simulink model "GPI1"  (Simulink 7.0)
settings: Solver=ode45  StartTime=0.0  StopTime=1000.0  RelTol=1e-3
values from neighbouring files (symbols this model uses):
  A_gpegpi = 1    [data_GPE.m]    (also in data_GPI.m)
  A_gpi = 2    [data_GPI.m]
  A_stngpi = 1    [data_GPI.m]    (also in data_STN.m)
  B_gpegpi = .1    (= 0.1)    [data_GPE.m]    (also in data_GPI.m)
  B_gpi = .08    (= 0.08)    [data_GPI.m]
  B_stngpi = .05    (= 0.05)    [data_GPI.m]    (also in data_STN.m)
  c_gpi = 1    [data_GPI.m]
  cagi0 = i_v_16(289:304)    [launch_sysGPI_mod.m]
  egpegpi = -100    [data_synapses.m]
  ek_gpi = -80.0    (= -80)    [data_GPI.m]
  el_gpi = -55.0    (= -55)    [data_GPI.m]
  epsil_gpi = 1*10^-4    (= 0.0001)    [data_GPI.m]
  estngpi = 0    [data_synapses.m]
  gahp_gpi = 30.0    (= 30)    [data_GPI.m]
  gca_gpi = 0.15    [data_GPI.m]
  ggpegpi = ggpegpi_vec(i)    [CN_launch_CN_analyze_TAL2.m]    (also in data_synapses.m = 1; launch_sysGPI_mod.m = 0.3)
  gk_gpi = 30.0    (= 30)    [data_GPI.m]
  gl_gpi = .1    (= 0.1)    [data_GPI.m]
  gna_gpi = 120    [data_GPI.m]
  gstngpi = .3    (= 0.3)    [data_synapses.m]
  gt_gpi = .5    (= 0.5)    [data_GPI.m]
  hgi0 = i_v_16(241:256)    [launch_sysGPI_mod.m]
  k1_gpi = 30.0    (= 30)    [data_GPI.m]
  kca_gpi = 15    [data_GPI.m]
  ngi0 = i_v_16(257:272)    [launch_sysGPI_mod.m]
  phih_gpi = 0.05    [data_GPI.m]
  phin_gpi = 0.1    [data_GPI.m]
  phir_gpi = 1    [data_GPI.m]
  rgi0 = i_v_16(273:288)    [launch_sysGPI_mod.m]
  sgi0 = i_v_16(305:320)    [launch_sysGPI_mod.m]
  sig0 = i_v_16(209:224)    [launch_sysGPI_mod.m]
  sigmaa_gpi = 2    [data_GPI.m]
  sigmagh_gpe = 2.0    (= 2)    [data_GPE.m]
  sigmagh_gpi = 2.0    (= 2)    [data_GPI.m]
  sigmagh_stn = 8.0    (= 8)    [data_STN.m]
  sigmah_gpi = -12    [data_GPI.m]
  sigmam_gpi = 10.0    (= 10)    [data_GPI.m]
  sigman_gpi = 14.0    (= 14)    [data_GPI.m]
  sigmar_gpi = -2.0    (= -2)    [data_GPI.m]
  sigmas_gpi = 2    [data_GPI.m]
  sigmatauh_gpi = -12    [data_GPI.m]
  sigmataun_gpi = -12.0    (= -12)    [data_GPI.m]
  sis0 = i_v_16(97:112)    [launch_sysGPI_mod.m]
  tauh0_gpi = .05    (= 0.05)    [data_GPI.m]
  tauh1_gpi = .27    (= 0.27)    [data_GPI.m]
  taun0_gpi = .05    (= 0.05)    [data_GPI.m]
  taun1_gpi = .27    (= 0.27)    [data_GPI.m]
  taur_gpi = 30.0    (= 30)    [data_GPI.m]
  theta_gpe = 20    [data_GPE.m]    (also in data_GPI.m)
  theta_gpi = 20    [data_GPI.m]
  theta_stn = 30    [data_GPI.m]    (also in data_STN.m)
  thetaa_gpi = -57.0    (= -57)    [data_GPI.m]
  thetagh_gpe = -57.0    (= -57)    [data_GPE.m]
  thetagh_gpi = -57.0    (= -57)    [data_GPI.m]
  thetagh_stn = -39.0    (= -39)    [data_STN.m]
  thetah_gpi = -58.0    (= -58)    [data_GPI.m]
  thetam_gpi = -37.0    (= -37)    [data_GPI.m]
  thetan_gpi = -50.0    (= -50)    [data_GPI.m]
  thetar_gpi = -70.0    (= -70)    [data_GPI.m]
  thetas_gpi = -35.0    (= -35)    [data_GPI.m]
  thetatauh_gpi = -40.0    (= -40)    [data_GPI.m]
  thetataun_gpi = -40.0    (= -40)    [data_GPI.m]
  vgi0 = i_v_16(225:240)    [launch_sysGPI_mod.m]
(part 2 of 6)

== system GPI1/gpicomp1/syn_gpegpi ==
  In1 : Inport  OutDataType=sfix(16)  OutScaling=2^0
  In2 : Inport  Port=2  OutDataType=sfix(16)  OutScaling=2^0
  Fcn : Fcn  Expr=1/(1+exp(-(u-theta_gpe-thetagh_gpe)/sigmagh_gpe))
  Fcn2 : Fcn  Orientation=left  Expr=A_gpegpi*(1-u)
  Gain : Gain  Orientation=left  Gain=B_gpegpi  ParameterDataType=sfix(16)  ParameterScaling=2^0  OutDataType=sfix(16)  OutScaling=2^0  SaturateOnIntegerOverflow=on
  Integrator : Integrator  InitialConditionSource=external
  Product : Product  OutDataType=sfix(16)  OutScaling=2^0  SaturateOnIntegerOverflow=on  InputSameDT=on
  Sum : Sum  Inputs=|+-  OutDataType=sfix(16)  OutScaling=2^0  SaturateOnIntegerOverflow=on  InputSameDT=on
  Out1 : Outport  OutDataType=sfix(16)  OutScaling=2^0
  wires:
  Fcn/1 -> Product/1
  Fcn2/1 -> Product/2
  Product/1 -> Sum/1
  Sum/1 -> Integrator/1
  Integrator/1 -> Gain/1, Fcn2/1, Out1/1
  Gain/1 -> Sum/2
  In1/1 -> Fcn/1
  In2/1 -> Integrator/2

== system GPI1/gpicomp1/syn_gpegpi1 ==
  In1 : Inport  OutDataType=sfix(16)  OutScaling=2^0
  In2 : Inport  Port=2  OutDataType=sfix(16)  OutScaling=2^0
  Fcn : Fcn  Expr=1/(1+exp(-(u-theta_gpi-thetagh_gpi)/sigmagh_gpi))
  Fcn2 : Fcn  Orientation=left  Expr=A_gpi*(1-u)
  Gain : Gain  Orientation=left  Gain=B_gpi  ParameterDataType=sfix(16)  ParameterScaling=2^0  OutDataType=sfix(16)  OutScaling=2^0  SaturateOnIntegerOverflow=on
  Integrator : Integrator  InitialConditionSource=external
  Product : Product  OutDataType=sfix(16)  OutScaling=2^0  SaturateOnIntegerOverflow=on  InputSameDT=on
  Sum : Sum  Inputs=|+-  OutDataType=sfix(16)  OutScaling=2^0  SaturateOnIntegerOverflow=on  InputSameDT=on
  Out1 : Outport  OutDataType=sfix(16)  OutScaling=2^0
  wires:
  Fcn/1 -> Product/1
  Fcn2/1 -> Product/2
  Product/1 -> Sum/1
  Sum/1 -> Integrator/1
  Integrator/1 -> Gain/1, Fcn2/1, Out1/1
  Gain/1 -> Sum/2
  In1/1 -> Fcn/1
  In2/1 -> Integrator/2

== system GPI1/gpicomp1/syn_stngpi ==
  In1 : Inport  OutDataType=sfix(16)  OutScaling=2^0
  In2 : Inport  Port=2  OutDataType=sfix(16)  OutScaling=2^0
  Fcn : Fcn  Expr=1/(1+exp(-(u-theta_stn-thetagh_stn)/sigmagh_stn))
  Fcn2 : Fcn  Orientation=left  Expr=A_stngpi*(1-u)
  Gain : Gain  Orientation=left  Gain=B_stngpi  ParameterDataType=sfix(16)  ParameterScaling=2^0  OutDataType=sfix(16)  OutScaling=2^0  SaturateOnIntegerOverflow=on
  Integrator : Integrator  InitialConditionSource=external
  Product : Product  OutDataType=sfix(16)  OutScaling=2^0  SaturateOnIntegerOverflow=on  InputSameDT=on
  Sum : Sum  Inputs=|+-  OutDataType=sfix(16)  OutScaling=2^0  SaturateOnIntegerOverflow=on  InputSameDT=on
  Out1 : Outport  OutDataType=sfix(16)  OutScaling=2^0
  wires:
  Fcn/1 -> Product/1
  Fcn2/1 -> Product/2
  Product/1 -> Sum/1
  Sum/1 -> Integrator/1
  Integrator/1 -> Gain/1, Fcn2/1, Out1/1
  Gain/1 -> Sum/2
  In1/1 -> Fcn/1
  In2/1 -> Integrator/2

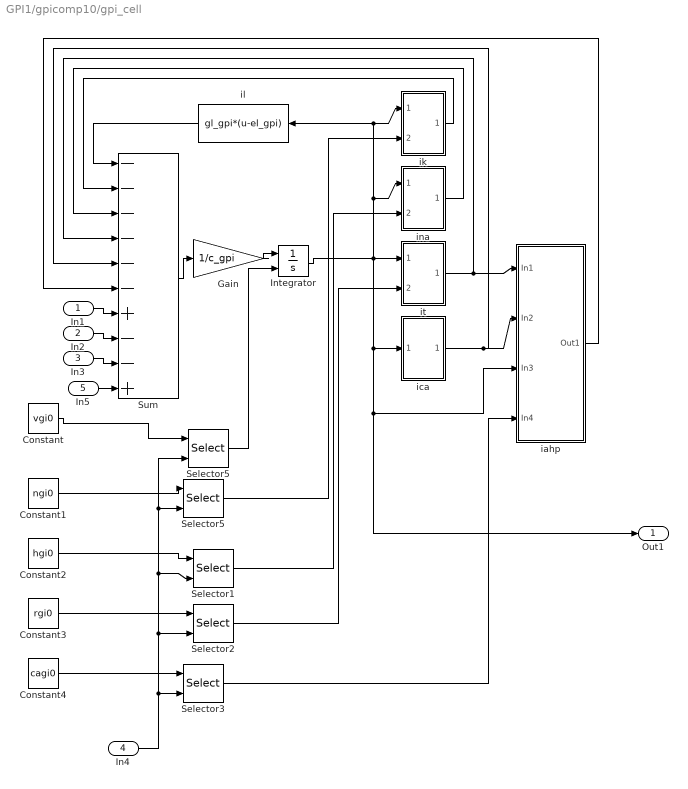
== system GPI1/gpicomp10/gpi_cell ==
  In1 : Inport  OutDataType=sfix(16)  OutScaling=2^0
  In2 : Inport  Port=2  OutDataType=sfix(16)  OutScaling=2^0
  In3 : Inport  Port=3  OutDataType=sfix(16)  OutScaling=2^0
  In4 : Inport  Port=4  OutDataType=sfix(16)  OutScaling=2^0
  In5 : Inport  Port=5  OutDataType=sfix(16)  OutScaling=2^0
  Constant : Constant  Value=vgi0  OutDataType=sfix(16)  OutScaling=2^0
  Constant1 : Constant  Value=ngi0  OutDataType=sfix(16)  OutScaling=2^0
  Constant2 : Constant  Value=hgi0  OutDataType=sfix(16)  OutScaling=2^0
  Constant3 : Constant  Value=rgi0  OutDataType=sfix(16)  OutScaling=2^0
  Constant4 : Constant  Value=cagi0  OutDataType=sfix(16)  OutScaling=2^0
  Gain : Gain  Gain=1/c_gpi  ParameterDataType=sfix(16)  ParameterScaling=2^0  OutDataType=sfix(16)  OutScaling=2^0  SaturateOnIntegerOverflow=on
  Integrator : Integrator  InitialConditionSource=external  InitialCondition=-67  LimitOutput=on  UpperSaturationLimit=80
  Selector{1..3,5} (4 alike) : Selector  IndexMode=Zero-based  IndexOptions=Index vector (port)  Indices=[1 3]  OutputSizes=1
  "Selector5 " : Selector  IndexMode=Zero-based  IndexOptions=Index vector (port)  Indices=[1 3]  OutputSizes=1
  Sum : Sum  Description=--------  Inputs=------+--+  OutDataType=sfix(16)  OutScaling=2^0  SaturateOnIntegerOverflow=on  InputSameDT=on
  iahp : Subsystem
  ica : Subsystem
  ik : Subsystem
  il : Fcn  Orientation=left  Expr=gl_gpi*(u-el_gpi)
  ina : Subsystem
  it : Subsystem
  Out1 : Outport  OutDataType=sfix(16)  OutScaling=2^0
  wires:
  Gain/1 -> Integrator/1
  Sum/1 -> Gain/1
  Integrator/1 -> il/1, ik/1(In1), ina/1(In2), it/1(In2), ica/1(In1), iahp/3(In3), Out1/1
  il/1 -> Sum/1
  ik/1(Out1) -> Sum/2
  ina/1(Out1) -> Sum/3
  ica/1(Out1) -> iahp/2(In2), Sum/5
  it/1(Out1) -> iahp/1(In1), Sum/4
  iahp/1(Out1) -> Sum/6
  In1/1 -> Sum/7
  In2/1 -> Sum/8
  In3/1 -> Sum/9
  "Selector5 "/1 -> Integrator/2
  Selector5/1 -> ik/2(In2)
  Selector1/1 -> ina/2(In1)
  Selector2/1 -> it/2(In1)
  Selector3/1 -> iahp/4(In4)
  In4/1 -> "Selector5 "/2, Selector5/2, Selector1/2, Selector2/2, Selector3/2
  Constant/1 -> "Selector5 "/1
  Constant1/1 -> Selector5/1
  Constant2/1 -> Selector1/1
  Constant3/1 -> Selector2/1
  Constant4/1 -> Selector3/1
  In5/1 -> Sum/10

== system GPI1/gpicomp10/igpegpi ==
  In1 : Inport  OutDataType=sfix(16)  OutScaling=2^0
  In3 : Inport  Port=2  OutDataType=sfix(16)  OutScaling=2^0
  Fcn : Fcn  Expr=ggpegpi*(u-egpegpi)
  Product : Product  OutDataType=sfix(16)  OutScaling=2^0  SaturateOnIntegerOverflow=on  InputSameDT=on
  Out1 : Outport  OutDataType=sfix(16)  OutScaling=2^0
  wires:
  Fcn/1 -> Product/2
  In1/1 -> Product/1
  Product/1 -> Out1/1
  In3/1 -> Fcn/1

== system GPI1/gpicomp10/istngpi ==
  In1 : Inport  OutDataType=sfix(16)  OutScaling=2^0
  In3 : Inport  Port=2  OutDataType=sfix(16)  OutScaling=2^0
  Fcn : Fcn  Expr=gstngpi*(u-estngpi)
  Product : Product  OutDataType=sfix(16)  OutScaling=2^0  SaturateOnIntegerOverflow=on  InputSameDT=on
  Out1 : Outport  OutDataType=sfix(16)  OutScaling=2^0
  wires:
  Fcn/1 -> Product/2
  In1/1 -> Product/1
  Product/1 -> Out1/1
  In3/1 -> Fcn/1

== system GPI1/gpicomp10/syn_gpegpi ==
  In1 : Inport  OutDataType=sfix(16)  OutScaling=2^0
  In2 : Inport  Port=2  OutDataType=sfix(16)  OutScaling=2^0
  Fcn : Fcn  Expr=1/(1+exp(-(u-theta_gpe-thetagh_gpe)/sigmagh_gpe))
  Fcn2 : Fcn  Orientation=left  Expr=A_gpegpi*(1-u)
  Gain : Gain  Orientation=left  Gain=B_gpegpi  ParameterDataType=sfix(16)  ParameterScaling=2^0  OutDataType=sfix(16)  OutScaling=2^0  SaturateOnIntegerOverflow=on
  Integrator : Integrator  InitialConditionSource=external
  Product : Product  OutDataType=sfix(16)  OutScaling=2^0  SaturateOnIntegerOverflow=on  InputSameDT=on
  Sum : Sum  Inputs=|+-  OutDataType=sfix(16)  OutScaling=2^0  SaturateOnIntegerOverflow=on  InputSameDT=on
  Out1 : Outport  OutDataType=sfix(16)  OutScaling=2^0
  wires:
  Fcn/1 -> Product/1
  Fcn2/1 -> Product/2
  Product/1 -> Sum/1
  Sum/1 -> Integrator/1
  Integrator/1 -> Gain/1, Fcn2/1, Out1/1
  Gain/1 -> Sum/2
  In1/1 -> Fcn/1
  In2/1 -> Integrator/2

== system GPI1/gpicomp10/syn_gpegpi1 ==
  In1 : Inport  OutDataType=sfix(16)  OutScaling=2^0
  In2 : Inport  Port=2  OutDataType=sfix(16)  OutScaling=2^0
  Fcn : Fcn  Expr=1/(1+exp(-(u-theta_gpi-thetagh_gpi)/sigmagh_gpi))
  Fcn2 : Fcn  Orientation=left  Expr=A_gpi*(1-u)
  Gain : Gain  Orientation=left  Gain=B_gpi  ParameterDataType=sfix(16)  ParameterScaling=2^0  OutDataType=sfix(16)  OutScaling=2^0  SaturateOnIntegerOverflow=on
  Integrator : Integrator  InitialConditionSource=external
  Product : Product  OutDataType=sfix(16)  OutScaling=2^0  SaturateOnIntegerOverflow=on  InputSameDT=on
  Sum : Sum  Inputs=|+-  OutDataType=sfix(16)  OutScaling=2^0  SaturateOnIntegerOverflow=on  InputSameDT=on
  Out1 : Outport  OutDataType=sfix(16)  OutScaling=2^0
  wires:
  Fcn/1 -> Product/1
  Fcn2/1 -> Product/2
  Product/1 -> Sum/1
  Sum/1 -> Integrator/1
  Integrator/1 -> Gain/1, Fcn2/1, Out1/1
  Gain/1 -> Sum/2
  In1/1 -> Fcn/1
  In2/1 -> Integrator/2

== system GPI1/gpicomp10/syn_stngpi ==
  In1 : Inport  OutDataType=sfix(16)  OutScaling=2^0
  In2 : Inport  Port=2  OutDataType=sfix(16)  OutScaling=2^0
  Fcn : Fcn  Expr=1/(1+exp(-(u-theta_stn-thetagh_stn)/sigmagh_stn))
  Fcn2 : Fcn  Orientation=left  Expr=A_stngpi*(1-u)
  Gain : Gain  Orientation=left  Gain=B_stngpi  ParameterDataType=sfix(16)  ParameterScaling=2^0  OutDataType=sfix(16)  OutScaling=2^0  SaturateOnIntegerOverflow=on
  Integrator : Integrator  InitialConditionSource=external
  Product : Product  OutDataType=sfix(16)  OutScaling=2^0  SaturateOnIntegerOverflow=on  InputSameDT=on
  Sum : Sum  Inputs=|+-  OutDataType=sfix(16)  OutScaling=2^0  SaturateOnIntegerOverflow=on  InputSameDT=on
  Out1 : Outport  OutDataType=sfix(16)  OutScaling=2^0
  wires:
  Fcn/1 -> Product/1
  Fcn2/1 -> Product/2
  Product/1 -> Sum/1
  Sum/1 -> Integrator/1
  Integrator/1 -> Gain/1, Fcn2/1, Out1/1
  Gain/1 -> Sum/2
  In1/1 -> Fcn/1
  In2/1 -> Integrator/2

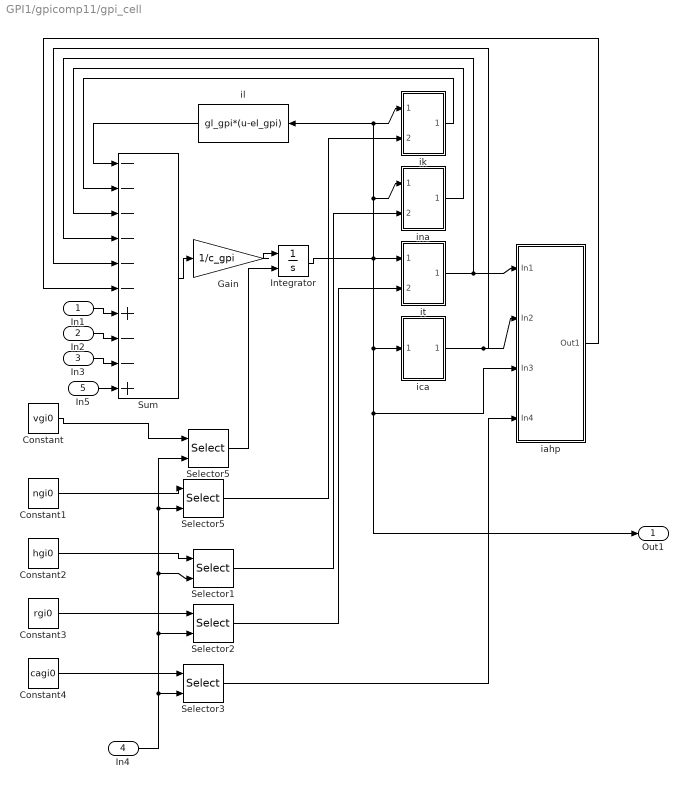
== system GPI1/gpicomp11/gpi_cell ==
  In1 : Inport  OutDataType=sfix(16)  OutScaling=2^0
  In2 : Inport  Port=2  OutDataType=sfix(16)  OutScaling=2^0
  In3 : Inport  Port=3  OutDataType=sfix(16)  OutScaling=2^0
  In4 : Inport  Port=4  OutDataType=sfix(16)  OutScaling=2^0
  In5 : Inport  Port=5  OutDataType=sfix(16)  OutScaling=2^0
  Constant : Constant  Value=vgi0  OutDataType=sfix(16)  OutScaling=2^0
  Constant1 : Constant  Value=ngi0  OutDataType=sfix(16)  OutScaling=2^0
  Constant2 : Constant  Value=hgi0  OutDataType=sfix(16)  OutScaling=2^0
  Constant3 : Constant  Value=rgi0  OutDataType=sfix(16)  OutScaling=2^0
  Constant4 : Constant  Value=cagi0  OutDataType=sfix(16)  OutScaling=2^0
  Gain : Gain  Gain=1/c_gpi  ParameterDataType=sfix(16)  ParameterScaling=2^0  OutDataType=sfix(16)  OutScaling=2^0  SaturateOnIntegerOverflow=on
  Integrator : Integrator  InitialConditionSource=external  InitialCondition=-67  LimitOutput=on  UpperSaturationLimit=80
  Selector{1..3,5} (4 alike) : Selector  IndexMode=Zero-based  IndexOptions=Index vector (port)  Indices=[1 3]  OutputSizes=1
  "Selector5 " : Selector  IndexMode=Zero-based  IndexOptions=Index vector (port)  Indices=[1 3]  OutputSizes=1
  Sum : Sum  Description=--------  Inputs=------+--+  OutDataType=sfix(16)  OutScaling=2^0  SaturateOnIntegerOverflow=on  InputSameDT=on
  iahp : Subsystem
  ica : Subsystem
  ik : Subsystem
  il : Fcn  Orientation=left  Expr=gl_gpi*(u-el_gpi)
  ina : Subsystem
  it : Subsystem
  Out1 : Outport  OutDataType=sfix(16)  OutScaling=2^0
  wires:
  Gain/1 -> Integrator/1
  Sum/1 -> Gain/1
  Integrator/1 -> il/1, ik/1(In1), ina/1(In2), it/1(In2), ica/1(In1), iahp/3(In3), Out1/1
  il/1 -> Sum/1
  ik/1(Out1) -> Sum/2
  ina/1(Out1) -> Sum/3
  ica/1(Out1) -> iahp/2(In2), Sum/5
  it/1(Out1) -> iahp/1(In1), Sum/4
  iahp/1(Out1) -> Sum/6
  In1/1 -> Sum/7
  In2/1 -> Sum/8
  In3/1 -> Sum/9
  "Selector5 "/1 -> Integrator/2
  Selector5/1 -> ik/2(In2)
  Selector1/1 -> ina/2(In1)
  Selector2/1 -> it/2(In1)
  Selector3/1 -> iahp/4(In4)
  In4/1 -> "Selector5 "/2, Selector5/2, Selector1/2, Selector2/2, Selector3/2
  Constant/1 -> "Selector5 "/1
  Constant1/1 -> Selector5/1
  Constant2/1 -> Selector1/1
  Constant3/1 -> Selector2/1
  Constant4/1 -> Selector3/1
  In5/1 -> Sum/10

== system GPI1/gpicomp11/igpegpi ==
  In1 : Inport  OutDataType=sfix(16)  OutScaling=2^0
  In3 : Inport  Port=2  OutDataType=sfix(16)  OutScaling=2^0
  Fcn : Fcn  Expr=ggpegpi*(u-egpegpi)
  Product : Product  OutDataType=sfix(16)  OutScaling=2^0  SaturateOnIntegerOverflow=on  InputSameDT=on
  Out1 : Outport  OutDataType=sfix(16)  OutScaling=2^0
  wires:
  Fcn/1 -> Product/2
  In1/1 -> Product/1
  Product/1 -> Out1/1
  In3/1 -> Fcn/1

== system GPI1/gpicomp11/istngpi ==
  In1 : Inport  OutDataType=sfix(16)  OutScaling=2^0
  In3 : Inport  Port=2  OutDataType=sfix(16)  OutScaling=2^0
  Fcn : Fcn  Expr=gstngpi*(u-estngpi)
  Product : Product  OutDataType=sfix(16)  OutScaling=2^0  SaturateOnIntegerOverflow=on  InputSameDT=on
  Out1 : Outport  OutDataType=sfix(16)  OutScaling=2^0
  wires:
  Fcn/1 -> Product/2
  In1/1 -> Product/1
  Product/1 -> Out1/1
  In3/1 -> Fcn/1

== system GPI1/gpicomp11/syn_gpegpi ==
  In1 : Inport  OutDataType=sfix(16)  OutScaling=2^0
  In2 : Inport  Port=2  OutDataType=sfix(16)  OutScaling=2^0
  Fcn : Fcn  Expr=1/(1+exp(-(u-theta_gpe-thetagh_gpe)/sigmagh_gpe))
  Fcn2 : Fcn  Orientation=left  Expr=A_gpegpi*(1-u)
  Gain : Gain  Orientation=left  Gain=B_gpegpi  ParameterDataType=sfix(16)  ParameterScaling=2^0  OutDataType=sfix(16)  OutScaling=2^0  SaturateOnIntegerOverflow=on
  Integrator : Integrator  InitialConditionSource=external
  Product : Product  OutDataType=sfix(16)  OutScaling=2^0  SaturateOnIntegerOverflow=on  InputSameDT=on
  Sum : Sum  Inputs=|+-  OutDataType=sfix(16)  OutScaling=2^0  SaturateOnIntegerOverflow=on  InputSameDT=on
  Out1 : Outport  OutDataType=sfix(16)  OutScaling=2^0
  wires:
  Fcn/1 -> Product/1
  Fcn2/1 -> Product/2
  Product/1 -> Sum/1
  Sum/1 -> Integrator/1
  Integrator/1 -> Gain/1, Fcn2/1, Out1/1
  Gain/1 -> Sum/2
  In1/1 -> Fcn/1
  In2/1 -> Integrator/2

== system GPI1/gpicomp11/syn_gpegpi1 ==
  In1 : Inport  OutDataType=sfix(16)  OutScaling=2^0
  In2 : Inport  Port=2  OutDataType=sfix(16)  OutScaling=2^0
  Fcn : Fcn  Expr=1/(1+exp(-(u-theta_gpi-thetagh_gpi)/sigmagh_gpi))
  Fcn2 : Fcn  Orientation=left  Expr=A_gpi*(1-u)
  Gain : Gain  Orientation=left  Gain=B_gpi  ParameterDataType=sfix(16)  ParameterScaling=2^0  OutDataType=sfix(16)  OutScaling=2^0  SaturateOnIntegerOverflow=on
  Integrator : Integrator  InitialConditionSource=external
  Product : Product  OutDataType=sfix(16)  OutScaling=2^0  SaturateOnIntegerOverflow=on  InputSameDT=on
  Sum : Sum  Inputs=|+-  OutDataType=sfix(16)  OutScaling=2^0  SaturateOnIntegerOverflow=on  InputSameDT=on
  Out1 : Outport  OutDataType=sfix(16)  OutScaling=2^0
  wires:
  Fcn/1 -> Product/1
  Fcn2/1 -> Product/2
  Product/1 -> Sum/1
  Sum/1 -> Integrator/1
  Integrator/1 -> Gain/1, Fcn2/1, Out1/1
  Gain/1 -> Sum/2
  In1/1 -> Fcn/1
  In2/1 -> Integrator/2

== system GPI1/gpicomp11/syn_stngpi ==
  In1 : Inport  OutDataType=sfix(16)  OutScaling=2^0
  In2 : Inport  Port=2  OutDataType=sfix(16)  OutScaling=2^0
  Fcn : Fcn  Expr=1/(1+exp(-(u-theta_stn-thetagh_stn)/sigmagh_stn))
  Fcn2 : Fcn  Orientation=left  Expr=A_stngpi*(1-u)
  Gain : Gain  Orientation=left  Gain=B_stngpi  ParameterDataType=sfix(16)  ParameterScaling=2^0  OutDataType=sfix(16)  OutScaling=2^0  SaturateOnIntegerOverflow=on
  Integrator : Integrator  InitialConditionSource=external
  Product : Product  OutDataType=sfix(16)  OutScaling=2^0  SaturateOnIntegerOverflow=on  InputSameDT=on
  Sum : Sum  Inputs=|+-  OutDataType=sfix(16)  OutScaling=2^0  SaturateOnIntegerOverflow=on  InputSameDT=on
  Out1 : Outport  OutDataType=sfix(16)  OutScaling=2^0
  wires:
  Fcn/1 -> Product/1
  Fcn2/1 -> Product/2
  Product/1 -> Sum/1
  Sum/1 -> Integrator/1
  Integrator/1 -> Gain/1, Fcn2/1, Out1/1
  Gain/1 -> Sum/2
  In1/1 -> Fcn/1
  In2/1 -> Integrator/2

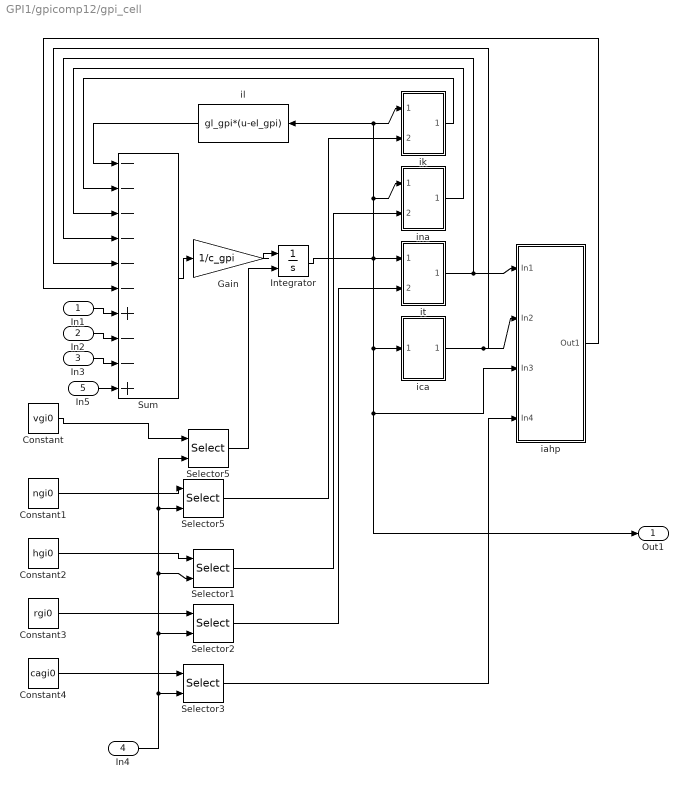
== system GPI1/gpicomp12/gpi_cell ==
  In1 : Inport  OutDataType=sfix(16)  OutScaling=2^0
  In2 : Inport  Port=2  OutDataType=sfix(16)  OutScaling=2^0
  In3 : Inport  Port=3  OutDataType=sfix(16)  OutScaling=2^0
  In4 : Inport  Port=4  OutDataType=sfix(16)  OutScaling=2^0
  In5 : Inport  Port=5  OutDataType=sfix(16)  OutScaling=2^0
  Constant : Constant  Value=vgi0  OutDataType=sfix(16)  OutScaling=2^0
  Constant1 : Constant  Value=ngi0  OutDataType=sfix(16)  OutScaling=2^0
  Constant2 : Constant  Value=hgi0  OutDataType=sfix(16)  OutScaling=2^0
  Constant3 : Constant  Value=rgi0  OutDataType=sfix(16)  OutScaling=2^0
  Constant4 : Constant  Value=cagi0  OutDataType=sfix(16)  OutScaling=2^0
  Gain : Gain  Gain=1/c_gpi  ParameterDataType=sfix(16)  ParameterScaling=2^0  OutDataType=sfix(16)  OutScaling=2^0  SaturateOnIntegerOverflow=on
  Integrator : Integrator  InitialConditionSource=external  InitialCondition=-67  LimitOutput=on  UpperSaturationLimit=80
  Selector{1..3,5} (4 alike) : Selector  IndexMode=Zero-based  IndexOptions=Index vector (port)  Indices=[1 3]  OutputSizes=1
  "Selector5 " : Selector  IndexMode=Zero-based  IndexOptions=Index vector (port)  Indices=[1 3]  OutputSizes=1
  Sum : Sum  Description=--------  Inputs=------+--+  OutDataType=sfix(16)  OutScaling=2^0  SaturateOnIntegerOverflow=on  InputSameDT=on
  iahp : Subsystem
  ica : Subsystem
  ik : Subsystem
  il : Fcn  Orientation=left  Expr=gl_gpi*(u-el_gpi)
  ina : Subsystem
  it : Subsystem
  Out1 : Outport  OutDataType=sfix(16)  OutScaling=2^0
  wires:
  Gain/1 -> Integrator/1
  Sum/1 -> Gain/1
  Integrator/1 -> il/1, ik/1(In1), ina/1(In2), it/1(In2), ica/1(In1), iahp/3(In3), Out1/1
  il/1 -> Sum/1
  ik/1(Out1) -> Sum/2
  ina/1(Out1) -> Sum/3
  ica/1(Out1) -> iahp/2(In2), Sum/5
  it/1(Out1) -> iahp/1(In1), Sum/4
  iahp/1(Out1) -> Sum/6
  In1/1 -> Sum/7
  In2/1 -> Sum/8
  In3/1 -> Sum/9
  "Selector5 "/1 -> Integrator/2
  Selector5/1 -> ik/2(In2)
  Selector1/1 -> ina/2(In1)
  Selector2/1 -> it/2(In1)
  Selector3/1 -> iahp/4(In4)
  In4/1 -> "Selector5 "/2, Selector5/2, Selector1/2, Selector2/2, Selector3/2
  Constant/1 -> "Selector5 "/1
  Constant1/1 -> Selector5/1
  Constant2/1 -> Selector1/1
  Constant3/1 -> Selector2/1
  Constant4/1 -> Selector3/1
  In5/1 -> Sum/10

== system GPI1/gpicomp12/igpegpi ==
  In1 : Inport  OutDataType=sfix(16)  OutScaling=2^0
  In3 : Inport  Port=2  OutDataType=sfix(16)  OutScaling=2^0
  Fcn : Fcn  Expr=ggpegpi*(u-egpegpi)
  Product : Product  OutDataType=sfix(16)  OutScaling=2^0  SaturateOnIntegerOverflow=on  InputSameDT=on
  Out1 : Outport  OutDataType=sfix(16)  OutScaling=2^0
  wires:
  Fcn/1 -> Product/2
  In1/1 -> Product/1
  Product/1 -> Out1/1
  In3/1 -> Fcn/1

== system GPI1/gpicomp12/istngpi ==
  In1 : Inport  OutDataType=sfix(16)  OutScaling=2^0
  In3 : Inport  Port=2  OutDataType=sfix(16)  OutScaling=2^0
  Fcn : Fcn  Expr=gstngpi*(u-estngpi)
  Product : Product  OutDataType=sfix(16)  OutScaling=2^0  SaturateOnIntegerOverflow=on  InputSameDT=on
  Out1 : Outport  OutDataType=sfix(16)  OutScaling=2^0
  wires:
  Fcn/1 -> Product/2
  In1/1 -> Product/1
  Product/1 -> Out1/1
  In3/1 -> Fcn/1

== system GPI1/gpicomp12/syn_gpegpi ==
  In1 : Inport  OutDataType=sfix(16)  OutScaling=2^0
  In2 : Inport  Port=2  OutDataType=sfix(16)  OutScaling=2^0
  Fcn : Fcn  Expr=1/(1+exp(-(u-theta_gpe-thetagh_gpe)/sigmagh_gpe))
  Fcn2 : Fcn  Orientation=left  Expr=A_gpegpi*(1-u)
  Gain : Gain  Orientation=left  Gain=B_gpegpi  ParameterDataType=sfix(16)  ParameterScaling=2^0  OutDataType=sfix(16)  OutScaling=2^0  SaturateOnIntegerOverflow=on
  Integrator : Integrator  InitialConditionSource=external
  Product : Product  OutDataType=sfix(16)  OutScaling=2^0  SaturateOnIntegerOverflow=on  InputSameDT=on
  Sum : Sum  Inputs=|+-  OutDataType=sfix(16)  OutScaling=2^0  SaturateOnIntegerOverflow=on  InputSameDT=on
  Out1 : Outport  OutDataType=sfix(16)  OutScaling=2^0
  wires:
  Fcn/1 -> Product/1
  Fcn2/1 -> Product/2
  Product/1 -> Sum/1
  Sum/1 -> Integrator/1
  Integrator/1 -> Gain/1, Fcn2/1, Out1/1
  Gain/1 -> Sum/2
  In1/1 -> Fcn/1
  In2/1 -> Integrator/2

== system GPI1/gpicomp12/syn_gpegpi1 ==
  In1 : Inport  OutDataType=sfix(16)  OutScaling=2^0
  In2 : Inport  Port=2  OutDataType=sfix(16)  OutScaling=2^0
  Fcn : Fcn  Expr=1/(1+exp(-(u-theta_gpi-thetagh_gpi)/sigmagh_gpi))
  Fcn2 : Fcn  Orientation=left  Expr=A_gpi*(1-u)
  Gain : Gain  Orientation=left  Gain=B_gpi  ParameterDataType=sfix(16)  ParameterScaling=2^0  OutDataType=sfix(16)  OutScaling=2^0  SaturateOnIntegerOverflow=on
  Integrator : Integrator  InitialConditionSource=external
  Product : Product  OutDataType=sfix(16)  OutScaling=2^0  SaturateOnIntegerOverflow=on  InputSameDT=on
  Sum : Sum  Inputs=|+-  OutDataType=sfix(16)  OutScaling=2^0  SaturateOnIntegerOverflow=on  InputSameDT=on
  Out1 : Outport  OutDataType=sfix(16)  OutScaling=2^0
  wires:
  Fcn/1 -> Product/1
  Fcn2/1 -> Product/2
  Product/1 -> Sum/1
  Sum/1 -> Integrator/1
  Integrator/1 -> Gain/1, Fcn2/1, Out1/1
  Gain/1 -> Sum/2
  In1/1 -> Fcn/1
  In2/1 -> Integrator/2

== system GPI1/gpicomp12/syn_stngpi ==
  In1 : Inport  OutDataType=sfix(16)  OutScaling=2^0
  In2 : Inport  Port=2  OutDataType=sfix(16)  OutScaling=2^0
  Fcn : Fcn  Expr=1/(1+exp(-(u-theta_stn-thetagh_stn)/sigmagh_stn))
  Fcn2 : Fcn  Orientation=left  Expr=A_stngpi*(1-u)
  Gain : Gain  Orientation=left  Gain=B_stngpi  ParameterDataType=sfix(16)  ParameterScaling=2^0  OutDataType=sfix(16)  OutScaling=2^0  SaturateOnIntegerOverflow=on
  Integrator : Integrator  InitialConditionSource=external
  Product : Product  OutDataType=sfix(16)  OutScaling=2^0  SaturateOnIntegerOverflow=on  InputSameDT=on
  Sum : Sum  Inputs=|+-  OutDataType=sfix(16)  OutScaling=2^0  SaturateOnIntegerOverflow=on  InputSameDT=on
  Out1 : Outport  OutDataType=sfix(16)  OutScaling=2^0
  wires:
  Fcn/1 -> Product/1
  Fcn2/1 -> Product/2
  Product/1 -> Sum/1
  Sum/1 -> Integrator/1
  Integrator/1 -> Gain/1, Fcn2/1, Out1/1
  Gain/1 -> Sum/2
  In1/1 -> Fcn/1
  In2/1 -> Integrator/2

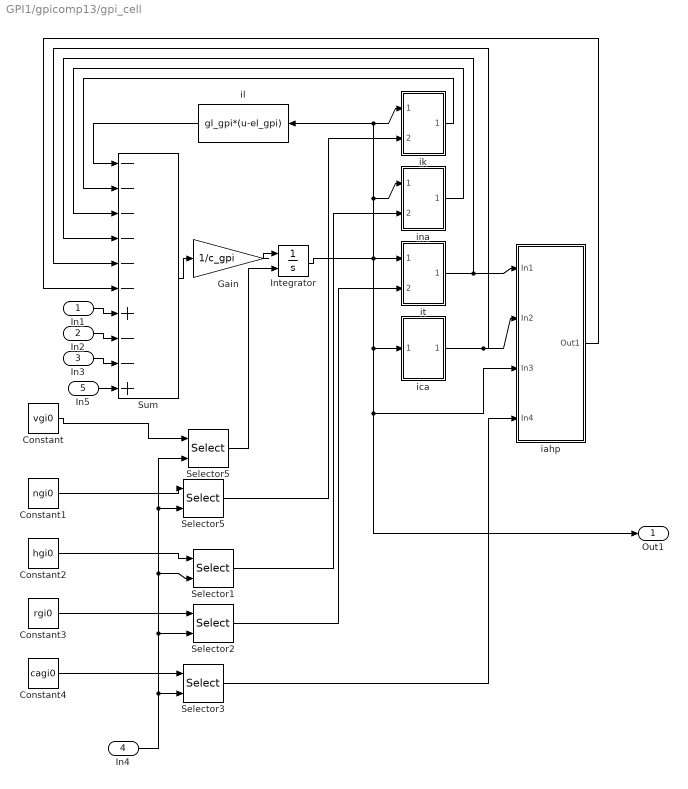
== system GPI1/gpicomp13/gpi_cell ==
  In1 : Inport  OutDataType=sfix(16)  OutScaling=2^0
  In2 : Inport  Port=2  OutDataType=sfix(16)  OutScaling=2^0
  In3 : Inport  Port=3  OutDataType=sfix(16)  OutScaling=2^0
  In4 : Inport  Port=4  OutDataType=sfix(16)  OutScaling=2^0
  In5 : Inport  Port=5  OutDataType=sfix(16)  OutScaling=2^0
  Constant : Constant  Value=vgi0  OutDataType=sfix(16)  OutScaling=2^0
  Constant1 : Constant  Value=ngi0  OutDataType=sfix(16)  OutScaling=2^0
  Constant2 : Constant  Value=hgi0  OutDataType=sfix(16)  OutScaling=2^0
  Constant3 : Constant  Value=rgi0  OutDataType=sfix(16)  OutScaling=2^0
  Constant4 : Constant  Value=cagi0  OutDataType=sfix(16)  OutScaling=2^0
  Gain : Gain  Gain=1/c_gpi  ParameterDataType=sfix(16)  ParameterScaling=2^0  OutDataType=sfix(16)  OutScaling=2^0  SaturateOnIntegerOverflow=on
  Integrator : Integrator  InitialConditionSource=external  InitialCondition=-67  LimitOutput=on  UpperSaturationLimit=80
  Selector{1..3,5} (4 alike) : Selector  IndexMode=Zero-based  IndexOptions=Index vector (port)  Indices=[1 3]  OutputSizes=1
  "Selector5 " : Selector  IndexMode=Zero-based  IndexOptions=Index vector (port)  Indices=[1 3]  OutputSizes=1
  Sum : Sum  Description=--------  Inputs=------+--+  OutDataType=sfix(16)  OutScaling=2^0  SaturateOnIntegerOverflow=on  InputSameDT=on
  iahp : Subsystem
  ica : Subsystem
  ik : Subsystem
  il : Fcn  Orientation=left  Expr=gl_gpi*(u-el_gpi)
  ina : Subsystem
  it : Subsystem
  Out1 : Outport  OutDataType=sfix(16)  OutScaling=2^0
  wires:
  Gain/1 -> Integrator/1
  Sum/1 -> Gain/1
  Integrator/1 -> il/1, ik/1(In1), ina/1(In2), it/1(In2), ica/1(In1), iahp/3(In3), Out1/1
  il/1 -> Sum/1
  ik/1(Out1) -> Sum/2
  ina/1(Out1) -> Sum/3
  ica/1(Out1) -> iahp/2(In2), Sum/5
  it/1(Out1) -> iahp/1(In1), Sum/4
  iahp/1(Out1) -> Sum/6
  In1/1 -> Sum/7
  In2/1 -> Sum/8
  In3/1 -> Sum/9
  "Selector5 "/1 -> Integrator/2
  Selector5/1 -> ik/2(In2)
  Selector1/1 -> ina/2(In1)
  Selector2/1 -> it/2(In1)
  Selector3/1 -> iahp/4(In4)
  In4/1 -> "Selector5 "/2, Selector5/2, Selector1/2, Selector2/2, Selector3/2
  Constant/1 -> "Selector5 "/1
  Constant1/1 -> Selector5/1
  Constant2/1 -> Selector1/1
  Constant3/1 -> Selector2/1
  Constant4/1 -> Selector3/1
  In5/1 -> Sum/10

== system GPI1/gpicomp13/igpegpi ==
  In1 : Inport  OutDataType=sfix(16)  OutScaling=2^0
  In3 : Inport  Port=2  OutDataType=sfix(16)  OutScaling=2^0
  Fcn : Fcn  Expr=ggpegpi*(u-egpegpi)
  Product : Product  OutDataType=sfix(16)  OutScaling=2^0  SaturateOnIntegerOverflow=on  InputSameDT=on
  Out1 : Outport  OutDataType=sfix(16)  OutScaling=2^0
  wires:
  Fcn/1 -> Product/2
  In1/1 -> Product/1
  Product/1 -> Out1/1
  In3/1 -> Fcn/1

== system GPI1/gpicomp13/istngpi ==
  In1 : Inport  OutDataType=sfix(16)  OutScaling=2^0
  In3 : Inport  Port=2  OutDataType=sfix(16)  OutScaling=2^0
  Fcn : Fcn  Expr=gstngpi*(u-estngpi)
  Product : Product  OutDataType=sfix(16)  OutScaling=2^0  SaturateOnIntegerOverflow=on  InputSameDT=on
  Out1 : Outport  OutDataType=sfix(16)  OutScaling=2^0
  wires:
  Fcn/1 -> Product/2
  In1/1 -> Product/1
  Product/1 -> Out1/1
  In3/1 -> Fcn/1

== system GPI1/gpicomp13/syn_gpegpi ==
  In1 : Inport  OutDataType=sfix(16)  OutScaling=2^0
  In2 : Inport  Port=2  OutDataType=sfix(16)  OutScaling=2^0
  Fcn : Fcn  Expr=1/(1+exp(-(u-theta_gpe-thetagh_gpe)/sigmagh_gpe))
  Fcn2 : Fcn  Orientation=left  Expr=A_gpegpi*(1-u)
  Gain : Gain  Orientation=left  Gain=B_gpegpi  ParameterDataType=sfix(16)  ParameterScaling=2^0  OutDataType=sfix(16)  OutScaling=2^0  SaturateOnIntegerOverflow=on
  Integrator : Integrator  InitialConditionSource=external
  Product : Product  OutDataType=sfix(16)  OutScaling=2^0  SaturateOnIntegerOverflow=on  InputSameDT=on
  Sum : Sum  Inputs=|+-  OutDataType=sfix(16)  OutScaling=2^0  SaturateOnIntegerOverflow=on  InputSameDT=on
  Out1 : Outport  OutDataType=sfix(16)  OutScaling=2^0
  wires:
  Fcn/1 -> Product/1
  Fcn2/1 -> Product/2
  Product/1 -> Sum/1
  Sum/1 -> Integrator/1
  Integrator/1 -> Gain/1, Fcn2/1, Out1/1
  Gain/1 -> Sum/2
  In1/1 -> Fcn/1
  In2/1 -> Integrator/2

== system GPI1/gpicomp13/syn_gpegpi1 ==
  In1 : Inport  OutDataType=sfix(16)  OutScaling=2^0
  In2 : Inport  Port=2  OutDataType=sfix(16)  OutScaling=2^0
  Fcn : Fcn  Expr=1/(1+exp(-(u-theta_gpi-thetagh_gpi)/sigmagh_gpi))
  Fcn2 : Fcn  Orientation=left  Expr=A_gpi*(1-u)
  Gain : Gain  Orientation=left  Gain=B_gpi  ParameterDataType=sfix(16)  ParameterScaling=2^0  OutDataType=sfix(16)  OutScaling=2^0  SaturateOnIntegerOverflow=on
  Integrator : Integrator  InitialConditionSource=external
  Product : Product  OutDataType=sfix(16)  OutScaling=2^0  SaturateOnIntegerOverflow=on  InputSameDT=on
  Sum : Sum  Inputs=|+-  OutDataType=sfix(16)  OutScaling=2^0  SaturateOnIntegerOverflow=on  InputSameDT=on
  Out1 : Outport  OutDataType=sfix(16)  OutScaling=2^0
  wires:
  Fcn/1 -> Product/1
  Fcn2/1 -> Product/2
  Product/1 -> Sum/1
  Sum/1 -> Integrator/1
  Integrator/1 -> Gain/1, Fcn2/1, Out1/1
  Gain/1 -> Sum/2
  In1/1 -> Fcn/1
  In2/1 -> Integrator/2

== system GPI1/gpicomp13/syn_stngpi ==
  In1 : Inport  OutDataType=sfix(16)  OutScaling=2^0
  In2 : Inport  Port=2  OutDataType=sfix(16)  OutScaling=2^0
  Fcn : Fcn  Expr=1/(1+exp(-(u-theta_stn-thetagh_stn)/sigmagh_stn))
  Fcn2 : Fcn  Orientation=left  Expr=A_stngpi*(1-u)
  Gain : Gain  Orientation=left  Gain=B_stngpi  ParameterDataType=sfix(16)  ParameterScaling=2^0  OutDataType=sfix(16)  OutScaling=2^0  SaturateOnIntegerOverflow=on
  Integrator : Integrator  InitialConditionSource=external
  Product : Product  OutDataType=sfix(16)  OutScaling=2^0  SaturateOnIntegerOverflow=on  InputSameDT=on
  Sum : Sum  Inputs=|+-  OutDataType=sfix(16)  OutScaling=2^0  SaturateOnIntegerOverflow=on  InputSameDT=on
  Out1 : Outport  OutDataType=sfix(16)  OutScaling=2^0
  wires:
  Fcn/1 -> Product/1
  Fcn2/1 -> Product/2
  Product/1 -> Sum/1
  Sum/1 -> Integrator/1
  Integrator/1 -> Gain/1, Fcn2/1, Out1/1
  Gain/1 -> Sum/2
  In1/1 -> Fcn/1
  In2/1 -> Integrator/2

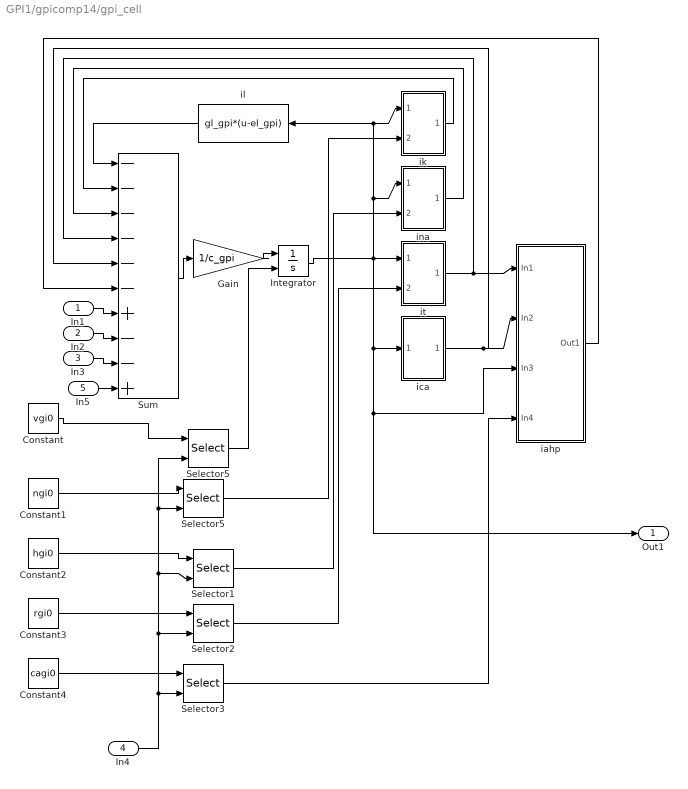
== system GPI1/gpicomp14/gpi_cell ==
  In1 : Inport  OutDataType=sfix(16)  OutScaling=2^0
  In2 : Inport  Port=2  OutDataType=sfix(16)  OutScaling=2^0
  In3 : Inport  Port=3  OutDataType=sfix(16)  OutScaling=2^0
  In4 : Inport  Port=4  OutDataType=sfix(16)  OutScaling=2^0
  In5 : Inport  Port=5  OutDataType=sfix(16)  OutScaling=2^0
  Constant : Constant  Value=vgi0  OutDataType=sfix(16)  OutScaling=2^0
  Constant1 : Constant  Value=ngi0  OutDataType=sfix(16)  OutScaling=2^0
  Constant2 : Constant  Value=hgi0  OutDataType=sfix(16)  OutScaling=2^0
  Constant3 : Constant  Value=rgi0  OutDataType=sfix(16)  OutScaling=2^0
  Constant4 : Constant  Value=cagi0  OutDataType=sfix(16)  OutScaling=2^0
  Gain : Gain  Gain=1/c_gpi  ParameterDataType=sfix(16)  ParameterScaling=2^0  OutDataType=sfix(16)  OutScaling=2^0  SaturateOnIntegerOverflow=on
  Integrator : Integrator  InitialConditionSource=external  InitialCondition=-67  LimitOutput=on  UpperSaturationLimit=80
  Selector{1..3,5} (4 alike) : Selector  IndexMode=Zero-based  IndexOptions=Index vector (port)  Indices=[1 3]  OutputSizes=1
  "Selector5 " : Selector  IndexMode=Zero-based  IndexOptions=Index vector (port)  Indices=[1 3]  OutputSizes=1
  Sum : Sum  Description=--------  Inputs=------+--+  OutDataType=sfix(16)  OutScaling=2^0  SaturateOnIntegerOverflow=on  InputSameDT=on
  iahp : Subsystem
  ica : Subsystem
  ik : Subsystem
  il : Fcn  Orientation=left  Expr=gl_gpi*(u-el_gpi)
  ina : Subsystem
  it : Subsystem
  Out1 : Outport  OutDataType=sfix(16)  OutScaling=2^0
  wires:
  Gain/1 -> Integrator/1
  Sum/1 -> Gain/1
  Integrator/1 -> il/1, ik/1(In1), ina/1(In2), it/1(In2), ica/1(In1), iahp/3(In3), Out1/1
  il/1 -> Sum/1
  ik/1(Out1) -> Sum/2
  ina/1(Out1) -> Sum/3
  ica/1(Out1) -> iahp/2(In2), Sum/5
  it/1(Out1) -> iahp/1(In1), Sum/4
  iahp/1(Out1) -> Sum/6
  In1/1 -> Sum/7
  In2/1 -> Sum/8
  In3/1 -> Sum/9
  "Selector5 "/1 -> Integrator/2
  Selector5/1 -> ik/2(In2)
  Selector1/1 -> ina/2(In1)
  Selector2/1 -> it/2(In1)
  Selector3/1 -> iahp/4(In4)
  In4/1 -> "Selector5 "/2, Selector5/2, Selector1/2, Selector2/2, Selector3/2
  Constant/1 -> "Selector5 "/1
  Constant1/1 -> Selector5/1
  Constant2/1 -> Selector1/1
  Constant3/1 -> Selector2/1
  Constant4/1 -> Selector3/1
  In5/1 -> Sum/10

== system GPI1/gpicomp14/igpegpi ==
  In1 : Inport  OutDataType=sfix(16)  OutScaling=2^0
  In3 : Inport  Port=2  OutDataType=sfix(16)  OutScaling=2^0
  Fcn : Fcn  Expr=ggpegpi*(u-egpegpi)
  Product : Product  OutDataType=sfix(16)  OutScaling=2^0  SaturateOnIntegerOverflow=on  InputSameDT=on
  Out1 : Outport  OutDataType=sfix(16)  OutScaling=2^0
  wires:
  Fcn/1 -> Product/2
  In1/1 -> Product/1
  Product/1 -> Out1/1
  In3/1 -> Fcn/1

== system GPI1/gpicomp14/istngpi ==
  In1 : Inport  OutDataType=sfix(16)  OutScaling=2^0
  In3 : Inport  Port=2  OutDataType=sfix(16)  OutScaling=2^0
  Fcn : Fcn  Expr=gstngpi*(u-estngpi)
  Product : Product  OutDataType=sfix(16)  OutScaling=2^0  SaturateOnIntegerOverflow=on  InputSameDT=on
  Out1 : Outport  OutDataType=sfix(16)  OutScaling=2^0
  wires:
  Fcn/1 -> Product/2
  In1/1 -> Product/1
  Product/1 -> Out1/1
  In3/1 -> Fcn/1

== system GPI1/gpicomp14/syn_gpegpi ==
  In1 : Inport  OutDataType=sfix(16)  OutScaling=2^0
  In2 : Inport  Port=2  OutDataType=sfix(16)  OutScaling=2^0
  Fcn : Fcn  Expr=1/(1+exp(-(u-theta_gpe-thetagh_gpe)/sigmagh_gpe))
  Fcn2 : Fcn  Orientation=left  Expr=A_gpegpi*(1-u)
  Gain : Gain  Orientation=left  Gain=B_gpegpi  ParameterDataType=sfix(16)  ParameterScaling=2^0  OutDataType=sfix(16)  OutScaling=2^0  SaturateOnIntegerOverflow=on
  Integrator : Integrator  InitialConditionSource=external
  Product : Product  OutDataType=sfix(16)  OutScaling=2^0  SaturateOnIntegerOverflow=on  InputSameDT=on
  Sum : Sum  Inputs=|+-  OutDataType=sfix(16)  OutScaling=2^0  SaturateOnIntegerOverflow=on  InputSameDT=on
  Out1 : Outport  OutDataType=sfix(16)  OutScaling=2^0
  wires:
  Fcn/1 -> Product/1
  Fcn2/1 -> Product/2
  Product/1 -> Sum/1
  Sum/1 -> Integrator/1
  Integrator/1 -> Gain/1, Fcn2/1, Out1/1
  Gain/1 -> Sum/2
  In1/1 -> Fcn/1
  In2/1 -> Integrator/2

== system GPI1/gpicomp14/syn_gpegpi1 ==
  In1 : Inport  OutDataType=sfix(16)  OutScaling=2^0
  In2 : Inport  Port=2  OutDataType=sfix(16)  OutScaling=2^0
  Fcn : Fcn  Expr=1/(1+exp(-(u-theta_gpi-thetagh_gpi)/sigmagh_gpi))
  Fcn2 : Fcn  Orientation=left  Expr=A_gpi*(1-u)
  Gain : Gain  Orientation=left  Gain=B_gpi  ParameterDataType=sfix(16)  ParameterScaling=2^0  OutDataType=sfix(16)  OutScaling=2^0  SaturateOnIntegerOverflow=on
  Integrator : Integrator  InitialConditionSource=external
  Product : Product  OutDataType=sfix(16)  OutScaling=2^0  SaturateOnIntegerOverflow=on  InputSameDT=on
  Sum : Sum  Inputs=|+-  OutDataType=sfix(16)  OutScaling=2^0  SaturateOnIntegerOverflow=on  InputSameDT=on
  Out1 : Outport  OutDataType=sfix(16)  OutScaling=2^0
  wires:
  Fcn/1 -> Product/1
  Fcn2/1 -> Product/2
  Product/1 -> Sum/1
  Sum/1 -> Integrator/1
  Integrator/1 -> Gain/1, Fcn2/1, Out1/1
  Gain/1 -> Sum/2
  In1/1 -> Fcn/1
  In2/1 -> Integrator/2

== system GPI1/gpicomp14/syn_stngpi ==
  In1 : Inport  OutDataType=sfix(16)  OutScaling=2^0
  In2 : Inport  Port=2  OutDataType=sfix(16)  OutScaling=2^0
  Fcn : Fcn  Expr=1/(1+exp(-(u-theta_stn-thetagh_stn)/sigmagh_stn))
  Fcn2 : Fcn  Orientation=left  Expr=A_stngpi*(1-u)
  Gain : Gain  Orientation=left  Gain=B_stngpi  ParameterDataType=sfix(16)  ParameterScaling=2^0  OutDataType=sfix(16)  OutScaling=2^0  SaturateOnIntegerOverflow=on
  Integrator : Integrator  InitialConditionSource=external
  Product : Product  OutDataType=sfix(16)  OutScaling=2^0  SaturateOnIntegerOverflow=on  InputSameDT=on
  Sum : Sum  Inputs=|+-  OutDataType=sfix(16)  OutScaling=2^0  SaturateOnIntegerOverflow=on  InputSameDT=on
  Out1 : Outport  OutDataType=sfix(16)  OutScaling=2^0
  wires:
  Fcn/1 -> Product/1
  Fcn2/1 -> Product/2
  Product/1 -> Sum/1
  Sum/1 -> Integrator/1
  Integrator/1 -> Gain/1, Fcn2/1, Out1/1
  Gain/1 -> Sum/2
  In1/1 -> Fcn/1
  In2/1 -> Integrator/2

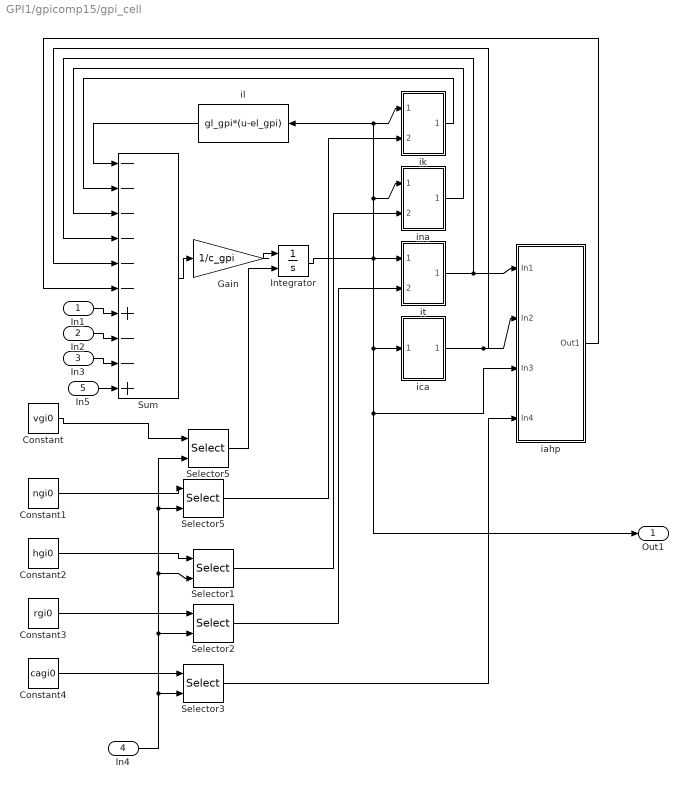
== system GPI1/gpicomp15/gpi_cell ==
  In1 : Inport  OutDataType=sfix(16)  OutScaling=2^0
  In2 : Inport  Port=2  OutDataType=sfix(16)  OutScaling=2^0
  In3 : Inport  Port=3  OutDataType=sfix(16)  OutScaling=2^0
  In4 : Inport  Port=4  OutDataType=sfix(16)  OutScaling=2^0
  In5 : Inport  Port=5  OutDataType=sfix(16)  OutScaling=2^0
  Constant : Constant  Value=vgi0  OutDataType=sfix(16)  OutScaling=2^0
  Constant1 : Constant  Value=ngi0  OutDataType=sfix(16)  OutScaling=2^0
  Constant2 : Constant  Value=hgi0  OutDataType=sfix(16)  OutScaling=2^0
  Constant3 : Constant  Value=rgi0  OutDataType=sfix(16)  OutScaling=2^0
  Constant4 : Constant  Value=cagi0  OutDataType=sfix(16)  OutScaling=2^0
  Gain : Gain  Gain=1/c_gpi  ParameterDataType=sfix(16)  ParameterScaling=2^0  OutDataType=sfix(16)  OutScaling=2^0  SaturateOnIntegerOverflow=on
  Integrator : Integrator  InitialConditionSource=external  InitialCondition=-67  LimitOutput=on  UpperSaturationLimit=80
  Selector{1..3,5} (4 alike) : Selector  IndexMode=Zero-based  IndexOptions=Index vector (port)  Indices=[1 3]  OutputSizes=1
  "Selector5 " : Selector  IndexMode=Zero-based  IndexOptions=Index vector (port)  Indices=[1 3]  OutputSizes=1
  Sum : Sum  Description=--------  Inputs=------+--+  OutDataType=sfix(16)  OutScaling=2^0  SaturateOnIntegerOverflow=on  InputSameDT=on
  iahp : Subsystem
  ica : Subsystem
  ik : Subsystem
  il : Fcn  Orientation=left  Expr=gl_gpi*(u-el_gpi)
  ina : Subsystem
  it : Subsystem
  Out1 : Outport  OutDataType=sfix(16)  OutScaling=2^0
  wires:
  Gain/1 -> Integrator/1
  Sum/1 -> Gain/1
  Integrator/1 -> il/1, ik/1(In1), ina/1(In2), it/1(In2), ica/1(In1), iahp/3(In3), Out1/1
  il/1 -> Sum/1
  ik/1(Out1) -> Sum/2
  ina/1(Out1) -> Sum/3
  ica/1(Out1) -> iahp/2(In2), Sum/5
  it/1(Out1) -> iahp/1(In1), Sum/4
  iahp/1(Out1) -> Sum/6
  In1/1 -> Sum/7
  In2/1 -> Sum/8
  In3/1 -> Sum/9
  "Selector5 "/1 -> Integrator/2
  Selector5/1 -> ik/2(In2)
  Selector1/1 -> ina/2(In1)
  Selector2/1 -> it/2(In1)
  Selector3/1 -> iahp/4(In4)
  In4/1 -> "Selector5 "/2, Selector5/2, Selector1/2, Selector2/2, Selector3/2
  Constant/1 -> "Selector5 "/1
  Constant1/1 -> Selector5/1
  Constant2/1 -> Selector1/1
  Constant3/1 -> Selector2/1
  Constant4/1 -> Selector3/1
  In5/1 -> Sum/10

== system GPI1/gpicomp15/igpegpi ==
  In1 : Inport  OutDataType=sfix(16)  OutScaling=2^0
  In3 : Inport  Port=2  OutDataType=sfix(16)  OutScaling=2^0
  Fcn : Fcn  Expr=ggpegpi*(u-egpegpi)
  Product : Product  OutDataType=sfix(16)  OutScaling=2^0  SaturateOnIntegerOverflow=on  InputSameDT=on
  Out1 : Outport  OutDataType=sfix(16)  OutScaling=2^0
  wires:
  Fcn/1 -> Product/2
  In1/1 -> Product/1
  Product/1 -> Out1/1
  In3/1 -> Fcn/1

== system GPI1/gpicomp15/istngpi ==
  In1 : Inport  OutDataType=sfix(16)  OutScaling=2^0
  In3 : Inport  Port=2  OutDataType=sfix(16)  OutScaling=2^0
  Fcn : Fcn  Expr=gstngpi*(u-estngpi)
  Product : Product  OutDataType=sfix(16)  OutScaling=2^0  SaturateOnIntegerOverflow=on  InputSameDT=on
  Out1 : Outport  OutDataType=sfix(16)  OutScaling=2^0
  wires:
  Fcn/1 -> Product/2
  In1/1 -> Product/1
  Product/1 -> Out1/1
  In3/1 -> Fcn/1

== system GPI1/gpicomp15/syn_gpegpi ==
  In1 : Inport  OutDataType=sfix(16)  OutScaling=2^0
  In2 : Inport  Port=2  OutDataType=sfix(16)  OutScaling=2^0
  Fcn : Fcn  Expr=1/(1+exp(-(u-theta_gpe-thetagh_gpe)/sigmagh_gpe))
  Fcn2 : Fcn  Orientation=left  Expr=A_gpegpi*(1-u)
  Gain : Gain  Orientation=left  Gain=B_gpegpi  ParameterDataType=sfix(16)  ParameterScaling=2^0  OutDataType=sfix(16)  OutScaling=2^0  SaturateOnIntegerOverflow=on
  Integrator : Integrator  InitialConditionSource=external
  Product : Product  OutDataType=sfix(16)  OutScaling=2^0  SaturateOnIntegerOverflow=on  InputSameDT=on
  Sum : Sum  Inputs=|+-  OutDataType=sfix(16)  OutScaling=2^0  SaturateOnIntegerOverflow=on  InputSameDT=on
  Out1 : Outport  OutDataType=sfix(16)  OutScaling=2^0
  wires:
  Fcn/1 -> Product/1
  Fcn2/1 -> Product/2
  Product/1 -> Sum/1
  Sum/1 -> Integrator/1
  Integrator/1 -> Gain/1, Fcn2/1, Out1/1
  Gain/1 -> Sum/2
  In1/1 -> Fcn/1
  In2/1 -> Integrator/2

== system GPI1/gpicomp15/syn_gpegpi1 ==
  In1 : Inport  OutDataType=sfix(16)  OutScaling=2^0
  In2 : Inport  Port=2  OutDataType=sfix(16)  OutScaling=2^0
  Fcn : Fcn  Expr=1/(1+exp(-(u-theta_gpi-thetagh_gpi)/sigmagh_gpi))
  Fcn2 : Fcn  Orientation=left  Expr=A_gpi*(1-u)
  Gain : Gain  Orientation=left  Gain=B_gpi  ParameterDataType=sfix(16)  ParameterScaling=2^0  OutDataType=sfix(16)  OutScaling=2^0  SaturateOnIntegerOverflow=on
  Integrator : Integrator  InitialConditionSource=external
  Product : Product  OutDataType=sfix(16)  OutScaling=2^0  SaturateOnIntegerOverflow=on  InputSameDT=on
  Sum : Sum  Inputs=|+-  OutDataType=sfix(16)  OutScaling=2^0  SaturateOnIntegerOverflow=on  InputSameDT=on
  Out1 : Outport  OutDataType=sfix(16)  OutScaling=2^0
  wires:
  Fcn/1 -> Product/1
  Fcn2/1 -> Product/2
  Product/1 -> Sum/1
  Sum/1 -> Integrator/1
  Integrator/1 -> Gain/1, Fcn2/1, Out1/1
  Gain/1 -> Sum/2
  In1/1 -> Fcn/1
  In2/1 -> Integrator/2

== system GPI1/gpicomp15/syn_stngpi ==
  In1 : Inport  OutDataType=sfix(16)  OutScaling=2^0
  In2 : Inport  Port=2  OutDataType=sfix(16)  OutScaling=2^0
  Fcn : Fcn  Expr=1/(1+exp(-(u-theta_stn-thetagh_stn)/sigmagh_stn))
  Fcn2 : Fcn  Orientation=left  Expr=A_stngpi*(1-u)
  Gain : Gain  Orientation=left  Gain=B_stngpi  ParameterDataType=sfix(16)  ParameterScaling=2^0  OutDataType=sfix(16)  OutScaling=2^0  SaturateOnIntegerOverflow=on
  Integrator : Integrator  InitialConditionSource=external
  Product : Product  OutDataType=sfix(16)  OutScaling=2^0  SaturateOnIntegerOverflow=on  InputSameDT=on
  Sum : Sum  Inputs=|+-  OutDataType=sfix(16)  OutScaling=2^0  SaturateOnIntegerOverflow=on  InputSameDT=on
  Out1 : Outport  OutDataType=sfix(16)  OutScaling=2^0
  wires:
  Fcn/1 -> Product/1
  Fcn2/1 -> Product/2
  Product/1 -> Sum/1
  Sum/1 -> Integrator/1
  Integrator/1 -> Gain/1, Fcn2/1, Out1/1
  Gain/1 -> Sum/2
  In1/1 -> Fcn/1
  In2/1 -> Integrator/2

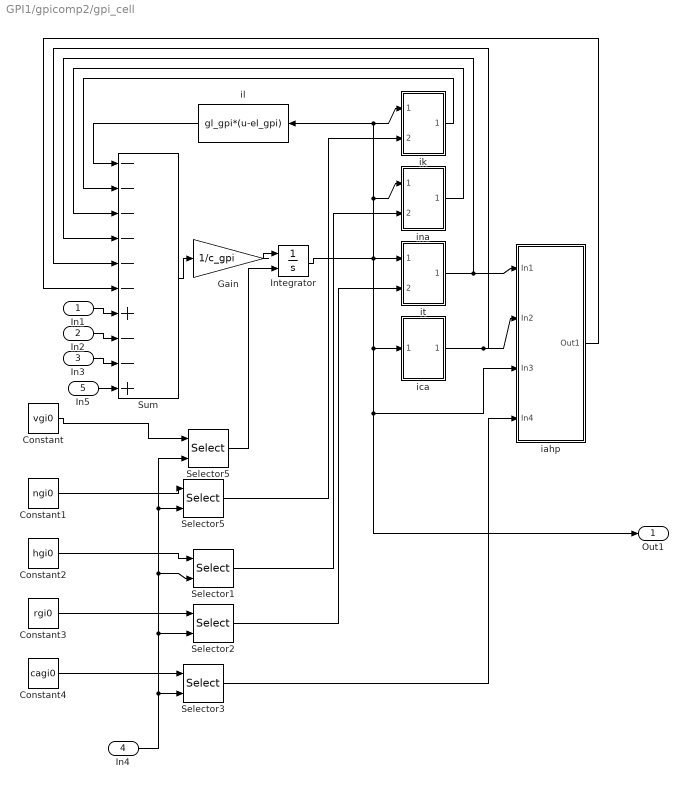
== system GPI1/gpicomp2/gpi_cell ==
  In1 : Inport  OutDataType=sfix(16)  OutScaling=2^0
  In2 : Inport  Port=2  OutDataType=sfix(16)  OutScaling=2^0
  In3 : Inport  Port=3  OutDataType=sfix(16)  OutScaling=2^0
  In4 : Inport  Port=4  OutDataType=sfix(16)  OutScaling=2^0
  In5 : Inport  Port=5  OutDataType=sfix(16)  OutScaling=2^0
  Constant : Constant  Value=vgi0  OutDataType=sfix(16)  OutScaling=2^0
  Constant1 : Constant  Value=ngi0  OutDataType=sfix(16)  OutScaling=2^0
  Constant2 : Constant  Value=hgi0  OutDataType=sfix(16)  OutScaling=2^0
  Constant3 : Constant  Value=rgi0  OutDataType=sfix(16)  OutScaling=2^0
  Constant4 : Constant  Value=cagi0  OutDataType=sfix(16)  OutScaling=2^0
  Gain : Gain  Gain=1/c_gpi  ParameterDataType=sfix(16)  ParameterScaling=2^0  OutDataType=sfix(16)  OutScaling=2^0  SaturateOnIntegerOverflow=on
  Integrator : Integrator  InitialConditionSource=external  InitialCondition=-67  LimitOutput=on  UpperSaturationLimit=80
  Selector{1..3,5} (4 alike) : Selector  IndexMode=Zero-based  IndexOptions=Index vector (port)  Indices=[1 3]  OutputSizes=1
  "Selector5 " : Selector  IndexMode=Zero-based  IndexOptions=Index vector (port)  Indices=[1 3]  OutputSizes=1
  Sum : Sum  Description=--------  Inputs=------+--+  OutDataType=sfix(16)  OutScaling=2^0  SaturateOnIntegerOverflow=on  InputSameDT=on
  iahp : Subsystem
  ica : Subsystem
  ik : Subsystem
  il : Fcn  Orientation=left  Expr=gl_gpi*(u-el_gpi)
  ina : Subsystem
  it : Subsystem
  Out1 : Outport  OutDataType=sfix(16)  OutScaling=2^0
  wires:
  Gain/1 -> Integrator/1
  Sum/1 -> Gain/1
  Integrator/1 -> il/1, ik/1(In1), ina/1(In2), it/1(In2), ica/1(In1), iahp/3(In3), Out1/1
  il/1 -> Sum/1
  ik/1(Out1) -> Sum/2
  ina/1(Out1) -> Sum/3
  ica/1(Out1) -> iahp/2(In2), Sum/5
  it/1(Out1) -> iahp/1(In1), Sum/4
  iahp/1(Out1) -> Sum/6
  In1/1 -> Sum/7
  In2/1 -> Sum/8
  In3/1 -> Sum/9
  "Selector5 "/1 -> Integrator/2
  Selector5/1 -> ik/2(In2)
  Selector1/1 -> ina/2(In1)
  Selector2/1 -> it/2(In1)
  Selector3/1 -> iahp/4(In4)
  In4/1 -> "Selector5 "/2, Selector5/2, Selector1/2, Selector2/2, Selector3/2
  Constant/1 -> "Selector5 "/1
  Constant1/1 -> Selector5/1
  Constant2/1 -> Selector1/1
  Constant3/1 -> Selector2/1
  Constant4/1 -> Selector3/1
  In5/1 -> Sum/10

== system GPI1/gpicomp2/igpegpi ==
  In1 : Inport  OutDataType=sfix(16)  OutScaling=2^0
  In3 : Inport  Port=2  OutDataType=sfix(16)  OutScaling=2^0
  Fcn : Fcn  Expr=ggpegpi*(u-egpegpi)
  Product : Product  OutDataType=sfix(16)  OutScaling=2^0  SaturateOnIntegerOverflow=on  InputSameDT=on
  Out1 : Outport  OutDataType=sfix(16)  OutScaling=2^0
  wires:
  Fcn/1 -> Product/2
  In1/1 -> Product/1
  Product/1 -> Out1/1
  In3/1 -> Fcn/1

== system GPI1/gpicomp2/istngpi ==
  In1 : Inport  OutDataType=sfix(16)  OutScaling=2^0
  In3 : Inport  Port=2  OutDataType=sfix(16)  OutScaling=2^0
  Fcn : Fcn  Expr=gstngpi*(u-estngpi)
  Product : Product  OutDataType=sfix(16)  OutScaling=2^0  SaturateOnIntegerOverflow=on  InputSameDT=on
  Out1 : Outport  OutDataType=sfix(16)  OutScaling=2^0
  wires:
  Fcn/1 -> Product/2
  In1/1 -> Product/1
  Product/1 -> Out1/1
  In3/1 -> Fcn/1

== system GPI1/gpicomp2/syn_gpegpi ==
  In1 : Inport  OutDataType=sfix(16)  OutScaling=2^0
  In2 : Inport  Port=2  OutDataType=sfix(16)  OutScaling=2^0
  Fcn : Fcn  Expr=1/(1+exp(-(u-theta_gpe-thetagh_gpe)/sigmagh_gpe))
  Fcn2 : Fcn  Orientation=left  Expr=A_gpegpi*(1-u)
  Gain : Gain  Orientation=left  Gain=B_gpegpi  ParameterDataType=sfix(16)  ParameterScaling=2^0  OutDataType=sfix(16)  OutScaling=2^0  SaturateOnIntegerOverflow=on
  Integrator : Integrator  InitialConditionSource=external
  Product : Product  OutDataType=sfix(16)  OutScaling=2^0  SaturateOnIntegerOverflow=on  InputSameDT=on
  Sum : Sum  Inputs=|+-  OutDataType=sfix(16)  OutScaling=2^0  SaturateOnIntegerOverflow=on  InputSameDT=on
  Out1 : Outport  OutDataType=sfix(16)  OutScaling=2^0
  wires:
  Fcn/1 -> Product/1
  Fcn2/1 -> Product/2
  Product/1 -> Sum/1
  Sum/1 -> Integrator/1
  Integrator/1 -> Gain/1, Fcn2/1, Out1/1
  Gain/1 -> Sum/2
  In1/1 -> Fcn/1
  In2/1 -> Integrator/2

== system GPI1/gpicomp2/syn_gpegpi1 ==
  In1 : Inport  OutDataType=sfix(16)  OutScaling=2^0
  In2 : Inport  Port=2  OutDataType=sfix(16)  OutScaling=2^0
  Fcn : Fcn  Expr=1/(1+exp(-(u-theta_gpi-thetagh_gpi)/sigmagh_gpi))
  Fcn2 : Fcn  Orientation=left  Expr=A_gpi*(1-u)
  Gain : Gain  Orientation=left  Gain=B_gpi  ParameterDataType=sfix(16)  ParameterScaling=2^0  OutDataType=sfix(16)  OutScaling=2^0  SaturateOnIntegerOverflow=on
  Integrator : Integrator  InitialConditionSource=external
  Product : Product  OutDataType=sfix(16)  OutScaling=2^0  SaturateOnIntegerOverflow=on  InputSameDT=on
  Sum : Sum  Inputs=|+-  OutDataType=sfix(16)  OutScaling=2^0  SaturateOnIntegerOverflow=on  InputSameDT=on
  Out1 : Outport  OutDataType=sfix(16)  OutScaling=2^0
  wires:
  Fcn/1 -> Product/1
  Fcn2/1 -> Product/2
  Product/1 -> Sum/1
  Sum/1 -> Integrator/1
  Integrator/1 -> Gain/1, Fcn2/1, Out1/1
  Gain/1 -> Sum/2
  In1/1 -> Fcn/1
  In2/1 -> Integrator/2

== system GPI1/gpicomp2/syn_stngpi ==
  In1 : Inport  OutDataType=sfix(16)  OutScaling=2^0
  In2 : Inport  Port=2  OutDataType=sfix(16)  OutScaling=2^0
  Fcn : Fcn  Expr=1/(1+exp(-(u-theta_stn-thetagh_stn)/sigmagh_stn))
  Fcn2 : Fcn  Orientation=left  Expr=A_stngpi*(1-u)
  Gain : Gain  Orientation=left  Gain=B_stngpi  ParameterDataType=sfix(16)  ParameterScaling=2^0  OutDataType=sfix(16)  OutScaling=2^0  SaturateOnIntegerOverflow=on
  Integrator : Integrator  InitialConditionSource=external
  Product : Product  OutDataType=sfix(16)  OutScaling=2^0  SaturateOnIntegerOverflow=on  InputSameDT=on
  Sum : Sum  Inputs=|+-  OutDataType=sfix(16)  OutScaling=2^0  SaturateOnIntegerOverflow=on  InputSameDT=on
  Out1 : Outport  OutDataType=sfix(16)  OutScaling=2^0
  wires:
  Fcn/1 -> Product/1
  Fcn2/1 -> Product/2
  Product/1 -> Sum/1
  Sum/1 -> Integrator/1
  Integrator/1 -> Gain/1, Fcn2/1, Out1/1
  Gain/1 -> Sum/2
  In1/1 -> Fcn/1
  In2/1 -> Integrator/2
